simulink model "StPassCmprtMd_RfCtrl_Sw_RclRspStat"  (R2018b)
settings: Solver=FixedStepDiscrete  StartTime=0.0  StopTime=10.0  FixedStep=0.01  RelTol=1e-3
undefined symbols (not defined in the file or in its folder): KeSMSuRspStatHldTm_Val, SrcReqTp1
libraries: RspLib x20
settings Model: Creator=sn2xws  LastModifiedBy=sn2xws
settings DataIOCC: SaveFormat=StructureWithTime
settings OptimizationCC: DefaultParameterBehavior=Inlined  EnhancedBackFolding=on  PassReuseOutputArgsAs=Individual arguments  ZeroExternalMemoryAtStartup=off  ZeroInternalMemoryAtStartup=off  OptimizeBlockOrder=speed  DifferentSizesBufferReuse=on  OptimizationCustomize=off
settings DebuggingCC: ParameterTunabilityLossMsg=error
settings ModelReferenceCC: ModelReferenceNumInstancesAllowed=Single
settings SFSimCC: MATLABDynamicMemAlloc=off
settings RTWCC: SystemTargetFile=autosar.tlc  GenCodeOnly=on  TemplateMakefile=ert_default_tmf  Description=AUTOSAR  GenerateReport=on  IncludeHyperlinkInReport=on  LaunchReport=on  GenerateTraceInfo=on  GenerateTraceReport=on  GenerateTraceReportSl=on  GenerateTraceReportSf=on  GenerateTraceReportEml=on
settings CodeAppCC: ForceParamTrailComments=on  IgnoreCustomStorageClasses=off  OperatorAnnotations=on  SimulinkDataObjDesc=on  SFDataObjDesc=on  InsertBlockDesc=on
settings STFCustomTargetCC: TargetLangStandard=C99 (ISO)  MultiwordLength=256  ParMdlRefBuildCompliant=on  CompOptLevelCompliant=on  IncludeMdlTerminateFcn=off  CombineOutputUpdateFcns=on  SuppressErrorStatus=on  ERTCustomFileBanners=on  SupportNonFinite=off  SupportComplex=off  SupportContinuousTime=off  SupportNonInlinedSFcns=off  RemoveResetFunc=on  MATLABClassNameForMDSCustomization=Simulink.SoftwareTarget.ERTCustomization  AutosarCompliant=on  UseToolchainInfoCompliant=on  LookupTableObjectStructAxisOrder=2,1,3,4,...  LUTObjectStructOrderEvenSpacing=Size,Table,Breakpoints  SystemTargetFile=autosar.tlc
settings ERTTargetCC: TargetLangStandard=C99 (ISO)  ConcurrentExecutionCompliant=off  IncludeMdlTerminateFcn=off  SuppressErrorStatus=on  SupportNonFinite=off  SupportComplex=off  ModelStepFunctionPrototypeControlCompliant=off  CPPClassGenCompliant=off  AutosarCompliant=on  LookupTableObjectStructAxisOrder=2,1,3,4,...  LUTObjectStructOrderEvenSpacing=Size,Table,Breakpoints  InlinedParameterPlacement=NonHierarchical  ERTCustomFileTemplate=example_file_process.tlc

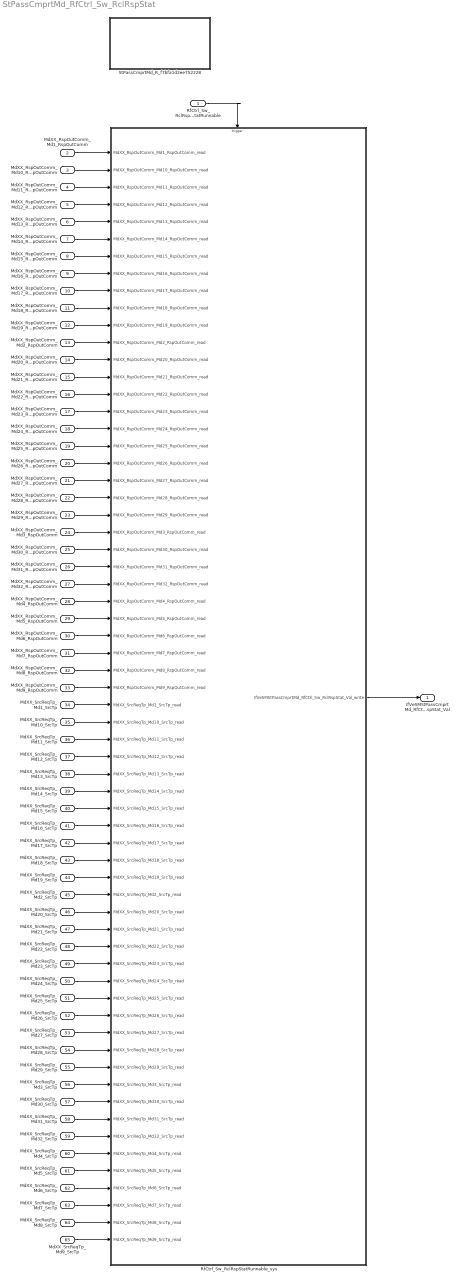
== system StPassCmprtMd_RfCtrl_Sw_RclRspStat ==
  RfCtrl_Sw_RclRspStatRunnable : Inport  SampleTime=0.01  OutputFunctionCall=on
  MdXX_RspOutComm_Md1_RspOutComm : Inport  Port=2  OutDataTypeStr=uint8  PortDimensions=1
  MdXX_RspOutComm_Md10_RspOutComm : Inport  Port=3  OutDataTypeStr=uint8  PortDimensions=1
  MdXX_RspOutComm_Md11_RspOutComm : Inport  Port=4  OutDataTypeStr=uint8  PortDimensions=1
  MdXX_RspOutComm_Md12_RspOutComm : Inport  Port=5  OutDataTypeStr=uint8  PortDimensions=1
  MdXX_RspOutComm_Md13_RspOutComm : Inport  Port=6  OutDataTypeStr=uint8  PortDimensions=1
  MdXX_RspOutComm_Md14_RspOutComm : Inport  Port=7  OutDataTypeStr=uint8  PortDimensions=1
  MdXX_RspOutComm_Md15_RspOutComm : Inport  Port=8  OutDataTypeStr=uint8  PortDimensions=1
  MdXX_RspOutComm_Md16_RspOutComm : Inport  Port=9  OutDataTypeStr=uint8  PortDimensions=1
  MdXX_RspOutComm_Md17_RspOutComm : Inport  Port=10  OutDataTypeStr=uint8  PortDimensions=1
  MdXX_RspOutComm_Md18_RspOutComm : Inport  Port=11  OutDataTypeStr=uint8  PortDimensions=1
  MdXX_RspOutComm_Md19_RspOutComm : Inport  Port=12  OutDataTypeStr=uint8  PortDimensions=1
  MdXX_RspOutComm_Md2_RspOutComm : Inport  Port=13  OutDataTypeStr=uint8  PortDimensions=1
  MdXX_RspOutComm_Md20_RspOutComm : Inport  Port=14  OutDataTypeStr=uint8  PortDimensions=1
  MdXX_RspOutComm_Md21_RspOutComm : Inport  Port=15  OutDataTypeStr=uint8  PortDimensions=1
  MdXX_RspOutComm_Md22_RspOutComm : Inport  Port=16  OutDataTypeStr=uint8  PortDimensions=1
  MdXX_RspOutComm_Md23_RspOutComm : Inport  Port=17  OutDataTypeStr=uint8  PortDimensions=1
  MdXX_RspOutComm_Md24_RspOutComm : Inport  Port=18  OutDataTypeStr=uint8  PortDimensions=1
  MdXX_RspOutComm_Md25_RspOutComm : Inport  Port=19  OutDataTypeStr=uint8  PortDimensions=1
  MdXX_RspOutComm_Md26_RspOutComm : Inport  Port=20  OutDataTypeStr=uint8  PortDimensions=1
  MdXX_RspOutComm_Md27_RspOutComm : Inport  Port=21  OutDataTypeStr=uint8  PortDimensions=1
  MdXX_RspOutComm_Md28_RspOutComm : Inport  Port=22  OutDataTypeStr=uint8  PortDimensions=1
  MdXX_RspOutComm_Md29_RspOutComm : Inport  Port=23  OutDataTypeStr=uint8  PortDimensions=1
  MdXX_RspOutComm_Md3_RspOutComm : Inport  Port=24  OutDataTypeStr=uint8  PortDimensions=1
  MdXX_RspOutComm_Md30_RspOutComm : Inport  Port=25  OutDataTypeStr=uint8  PortDimensions=1
  MdXX_RspOutComm_Md31_RspOutComm : Inport  Port=26  OutDataTypeStr=uint8  PortDimensions=1
  MdXX_RspOutComm_Md32_RspOutComm : Inport  Port=27  OutDataTypeStr=uint8  PortDimensions=1
  MdXX_RspOutComm_Md4_RspOutComm : Inport  Port=28  OutDataTypeStr=uint8  PortDimensions=1
  MdXX_RspOutComm_Md5_RspOutComm : Inport  Port=29  OutDataTypeStr=uint8  PortDimensions=1
  MdXX_RspOutComm_Md6_RspOutComm : Inport  Port=30  OutDataTypeStr=uint8  PortDimensions=1
  MdXX_RspOutComm_Md7_RspOutComm : Inport  Port=31  OutDataTypeStr=uint8  PortDimensions=1
  MdXX_RspOutComm_Md8_RspOutComm : Inport  Port=32  OutDataTypeStr=uint8  PortDimensions=1
  MdXX_RspOutComm_Md9_RspOutComm : Inport  Port=33  OutDataTypeStr=uint8  PortDimensions=1
  MdXX_SrcReqTp_Md1_SrcTp : Inport  Port=34  OutDataTypeStr=Enum: SrcReqTp1  PortDimensions=1
  MdXX_SrcReqTp_Md10_SrcTp : Inport  Port=35  OutDataTypeStr=Enum: SrcReqTp1  PortDimensions=1
  MdXX_SrcReqTp_Md11_SrcTp : Inport  Port=36  OutDataTypeStr=Enum: SrcReqTp1  PortDimensions=1
  MdXX_SrcReqTp_Md12_SrcTp : Inport  Port=37  OutDataTypeStr=Enum: SrcReqTp1  PortDimensions=1
  MdXX_SrcReqTp_Md13_SrcTp : Inport  Port=38  OutDataTypeStr=Enum: SrcReqTp1  PortDimensions=1
  MdXX_SrcReqTp_Md14_SrcTp : Inport  Port=39  OutDataTypeStr=Enum: SrcReqTp1  PortDimensions=1
  MdXX_SrcReqTp_Md15_SrcTp : Inport  Port=40  OutDataTypeStr=Enum: SrcReqTp1  PortDimensions=1
  MdXX_SrcReqTp_Md16_SrcTp : Inport  Port=41  OutDataTypeStr=Enum: SrcReqTp1  PortDimensions=1
  MdXX_SrcReqTp_Md17_SrcTp : Inport  Port=42  OutDataTypeStr=Enum: SrcReqTp1  PortDimensions=1
  MdXX_SrcReqTp_Md18_SrcTp : Inport  Port=43  OutDataTypeStr=Enum: SrcReqTp1  PortDimensions=1
  MdXX_SrcReqTp_Md19_SrcTp : Inport  Port=44  OutDataTypeStr=Enum: SrcReqTp1  PortDimensions=1
  MdXX_SrcReqTp_Md2_SrcTp : Inport  Port=45  OutDataTypeStr=Enum: SrcReqTp1  PortDimensions=1
  MdXX_SrcReqTp_Md20_SrcTp : Inport  Port=46  OutDataTypeStr=Enum: SrcReqTp1  PortDimensions=1
  MdXX_SrcReqTp_Md21_SrcTp : Inport  Port=47  OutDataTypeStr=Enum: SrcReqTp1  PortDimensions=1
  MdXX_SrcReqTp_Md22_SrcTp : Inport  Port=48  OutDataTypeStr=Enum: SrcReqTp1  PortDimensions=1
  MdXX_SrcReqTp_Md23_SrcTp : Inport  Port=49  OutDataTypeStr=Enum: SrcReqTp1  PortDimensions=1
  MdXX_SrcReqTp_Md24_SrcTp : Inport  Port=50  OutDataTypeStr=Enum: SrcReqTp1  PortDimensions=1
  MdXX_SrcReqTp_Md25_SrcTp : Inport  Port=51  OutDataTypeStr=Enum: SrcReqTp1  PortDimensions=1
  MdXX_SrcReqTp_Md26_SrcTp : Inport  Port=52  OutDataTypeStr=Enum: SrcReqTp1  PortDimensions=1
  MdXX_SrcReqTp_Md27_SrcTp : Inport  Port=53  OutDataTypeStr=Enum: SrcReqTp1  PortDimensions=1
  MdXX_SrcReqTp_Md28_SrcTp : Inport  Port=54  OutDataTypeStr=Enum: SrcReqTp1  PortDimensions=1
  MdXX_SrcReqTp_Md29_SrcTp : Inport  Port=55  OutDataTypeStr=Enum: SrcReqTp1  PortDimensions=1
  MdXX_SrcReqTp_Md3_SrcTp : Inport  Port=56  OutDataTypeStr=Enum: SrcReqTp1  PortDimensions=1
  MdXX_SrcReqTp_Md30_SrcTp : Inport  Port=57  OutDataTypeStr=Enum: SrcReqTp1  PortDimensions=1
  MdXX_SrcReqTp_Md31_SrcTp : Inport  Port=58  OutDataTypeStr=Enum: SrcReqTp1  PortDimensions=1
  MdXX_SrcReqTp_Md32_SrcTp : Inport  Port=59  OutDataTypeStr=Enum: SrcReqTp1  PortDimensions=1
  MdXX_SrcReqTp_Md4_SrcTp : Inport  Port=60  OutDataTypeStr=Enum: SrcReqTp1  PortDimensions=1
  MdXX_SrcReqTp_Md5_SrcTp : Inport  Port=61  OutDataTypeStr=Enum: SrcReqTp1  PortDimensions=1
  MdXX_SrcReqTp_Md6_SrcTp : Inport  Port=62  OutDataTypeStr=Enum: SrcReqTp1  PortDimensions=1
  MdXX_SrcReqTp_Md7_SrcTp : Inport  Port=63  OutDataTypeStr=Enum: SrcReqTp1  PortDimensions=1
  MdXX_SrcReqTp_Md8_SrcTp : Inport  Port=64  OutDataTypeStr=Enum: SrcReqTp1  PortDimensions=1
  MdXX_SrcReqTp_Md9_SrcTp : Inport  Port=65  OutDataTypeStr=Enum: SrcReqTp1  PortDimensions=1
  RfCtrl_Sw_RclRspStatRunnable_sys : Subsystem
  StPassCmprtMd_R_f7bfa1d2ee752228 : Subsystem
  IfVeSMStPassCmprtMd_RfCtrl_Sw_RclRspStat_Val : Outport  OutDataTypeStr=uint8  PortDimensions=1
  wires:
  MdXX_RspOutComm_Md1_RspOutComm/1 -> RfCtrl_Sw_RclRspStatRunnable_sys/1(MdXX_RspOutComm_Md1_RspOutComm_read)
  MdXX_RspOutComm_Md10_RspOutComm/1 -> RfCtrl_Sw_RclRspStatRunnable_sys/2(MdXX_RspOutComm_Md10_RspOutComm_read)
  MdXX_RspOutComm_Md11_RspOutComm/1 -> RfCtrl_Sw_RclRspStatRunnable_sys/3(MdXX_RspOutComm_Md11_RspOutComm_read)
  MdXX_RspOutComm_Md12_RspOutComm/1 -> RfCtrl_Sw_RclRspStatRunnable_sys/4(MdXX_RspOutComm_Md12_RspOutComm_read)
  MdXX_RspOutComm_Md13_RspOutComm/1 -> RfCtrl_Sw_RclRspStatRunnable_sys/5(MdXX_RspOutComm_Md13_RspOutComm_read)
  MdXX_RspOutComm_Md14_RspOutComm/1 -> RfCtrl_Sw_RclRspStatRunnable_sys/6(MdXX_RspOutComm_Md14_RspOutComm_read)
  MdXX_RspOutComm_Md15_RspOutComm/1 -> RfCtrl_Sw_RclRspStatRunnable_sys/7(MdXX_RspOutComm_Md15_RspOutComm_read)
  MdXX_RspOutComm_Md16_RspOutComm/1 -> RfCtrl_Sw_RclRspStatRunnable_sys/8(MdXX_RspOutComm_Md16_RspOutComm_read)
  MdXX_RspOutComm_Md17_RspOutComm/1 -> RfCtrl_Sw_RclRspStatRunnable_sys/9(MdXX_RspOutComm_Md17_RspOutComm_read)
  MdXX_RspOutComm_Md18_RspOutComm/1 -> RfCtrl_Sw_RclRspStatRunnable_sys/10(MdXX_RspOutComm_Md18_RspOutComm_read)
  MdXX_RspOutComm_Md19_RspOutComm/1 -> RfCtrl_Sw_RclRspStatRunnable_sys/11(MdXX_RspOutComm_Md19_RspOutComm_read)
  MdXX_RspOutComm_Md2_RspOutComm/1 -> RfCtrl_Sw_RclRspStatRunnable_sys/12(MdXX_RspOutComm_Md2_RspOutComm_read)
  MdXX_RspOutComm_Md20_RspOutComm/1 -> RfCtrl_Sw_RclRspStatRunnable_sys/13(MdXX_RspOutComm_Md20_RspOutComm_read)
  MdXX_RspOutComm_Md21_RspOutComm/1 -> RfCtrl_Sw_RclRspStatRunnable_sys/14(MdXX_RspOutComm_Md21_RspOutComm_read)
  MdXX_RspOutComm_Md22_RspOutComm/1 -> RfCtrl_Sw_RclRspStatRunnable_sys/15(MdXX_RspOutComm_Md22_RspOutComm_read)
  MdXX_RspOutComm_Md23_RspOutComm/1 -> RfCtrl_Sw_RclRspStatRunnable_sys/16(MdXX_RspOutComm_Md23_RspOutComm_read)
  MdXX_RspOutComm_Md24_RspOutComm/1 -> RfCtrl_Sw_RclRspStatRunnable_sys/17(MdXX_RspOutComm_Md24_RspOutComm_read)
  MdXX_RspOutComm_Md25_RspOutComm/1 -> RfCtrl_Sw_RclRspStatRunnable_sys/18(MdXX_RspOutComm_Md25_RspOutComm_read)
  MdXX_RspOutComm_Md26_RspOutComm/1 -> RfCtrl_Sw_RclRspStatRunnable_sys/19(MdXX_RspOutComm_Md26_RspOutComm_read)
  MdXX_RspOutComm_Md27_RspOutComm/1 -> RfCtrl_Sw_RclRspStatRunnable_sys/20(MdXX_RspOutComm_Md27_RspOutComm_read)
  MdXX_RspOutComm_Md28_RspOutComm/1 -> RfCtrl_Sw_RclRspStatRunnable_sys/21(MdXX_RspOutComm_Md28_RspOutComm_read)
  MdXX_RspOutComm_Md29_RspOutComm/1 -> RfCtrl_Sw_RclRspStatRunnable_sys/22(MdXX_RspOutComm_Md29_RspOutComm_read)
  MdXX_RspOutComm_Md3_RspOutComm/1 -> RfCtrl_Sw_RclRspStatRunnable_sys/23(MdXX_RspOutComm_Md3_RspOutComm_read)
  MdXX_RspOutComm_Md30_RspOutComm/1 -> RfCtrl_Sw_RclRspStatRunnable_sys/24(MdXX_RspOutComm_Md30_RspOutComm_read)
  MdXX_RspOutComm_Md31_RspOutComm/1 -> RfCtrl_Sw_RclRspStatRunnable_sys/25(MdXX_RspOutComm_Md31_RspOutComm_read)
  MdXX_RspOutComm_Md32_RspOutComm/1 -> RfCtrl_Sw_RclRspStatRunnable_sys/26(MdXX_RspOutComm_Md32_RspOutComm_read)
  MdXX_RspOutComm_Md4_RspOutComm/1 -> RfCtrl_Sw_RclRspStatRunnable_sys/27(MdXX_RspOutComm_Md4_RspOutComm_read)
  MdXX_RspOutComm_Md5_RspOutComm/1 -> RfCtrl_Sw_RclRspStatRunnable_sys/28(MdXX_RspOutComm_Md5_RspOutComm_read)
  MdXX_RspOutComm_Md6_RspOutComm/1 -> RfCtrl_Sw_RclRspStatRunnable_sys/29(MdXX_RspOutComm_Md6_RspOutComm_read)
  MdXX_RspOutComm_Md7_RspOutComm/1 -> RfCtrl_Sw_RclRspStatRunnable_sys/30(MdXX_RspOutComm_Md7_RspOutComm_read)
  MdXX_RspOutComm_Md8_RspOutComm/1 -> RfCtrl_Sw_RclRspStatRunnable_sys/31(MdXX_RspOutComm_Md8_RspOutComm_read)
  MdXX_RspOutComm_Md9_RspOutComm/1 -> RfCtrl_Sw_RclRspStatRunnable_sys/32(MdXX_RspOutComm_Md9_RspOutComm_read)
  MdXX_SrcReqTp_Md1_SrcTp/1 -> RfCtrl_Sw_RclRspStatRunnable_sys/33(MdXX_SrcReqTp_Md1_SrcTp_read)
  MdXX_SrcReqTp_Md10_SrcTp/1 -> RfCtrl_Sw_RclRspStatRunnable_sys/34(MdXX_SrcReqTp_Md10_SrcTp_read)
  MdXX_SrcReqTp_Md11_SrcTp/1 -> RfCtrl_Sw_RclRspStatRunnable_sys/35(MdXX_SrcReqTp_Md11_SrcTp_read)
  MdXX_SrcReqTp_Md12_SrcTp/1 -> RfCtrl_Sw_RclRspStatRunnable_sys/36(MdXX_SrcReqTp_Md12_SrcTp_read)
  MdXX_SrcReqTp_Md13_SrcTp/1 -> RfCtrl_Sw_RclRspStatRunnable_sys/37(MdXX_SrcReqTp_Md13_SrcTp_read)
  MdXX_SrcReqTp_Md14_SrcTp/1 -> RfCtrl_Sw_RclRspStatRunnable_sys/38(MdXX_SrcReqTp_Md14_SrcTp_read)
  MdXX_SrcReqTp_Md15_SrcTp/1 -> RfCtrl_Sw_RclRspStatRunnable_sys/39(MdXX_SrcReqTp_Md15_SrcTp_read)
  MdXX_SrcReqTp_Md16_SrcTp/1 -> RfCtrl_Sw_RclRspStatRunnable_sys/40(MdXX_SrcReqTp_Md16_SrcTp_read)
  MdXX_SrcReqTp_Md17_SrcTp/1 -> RfCtrl_Sw_RclRspStatRunnable_sys/41(MdXX_SrcReqTp_Md17_SrcTp_read)
  MdXX_SrcReqTp_Md18_SrcTp/1 -> RfCtrl_Sw_RclRspStatRunnable_sys/42(MdXX_SrcReqTp_Md18_SrcTp_read)
  MdXX_SrcReqTp_Md19_SrcTp/1 -> RfCtrl_Sw_RclRspStatRunnable_sys/43(MdXX_SrcReqTp_Md19_SrcTp_read)
  MdXX_SrcReqTp_Md2_SrcTp/1 -> RfCtrl_Sw_RclRspStatRunnable_sys/44(MdXX_SrcReqTp_Md2_SrcTp_read)
  MdXX_SrcReqTp_Md20_SrcTp/1 -> RfCtrl_Sw_RclRspStatRunnable_sys/45(MdXX_SrcReqTp_Md20_SrcTp_read)
  MdXX_SrcReqTp_Md21_SrcTp/1 -> RfCtrl_Sw_RclRspStatRunnable_sys/46(MdXX_SrcReqTp_Md21_SrcTp_read)
  MdXX_SrcReqTp_Md22_SrcTp/1 -> RfCtrl_Sw_RclRspStatRunnable_sys/47(MdXX_SrcReqTp_Md22_SrcTp_read)
  MdXX_SrcReqTp_Md23_SrcTp/1 -> RfCtrl_Sw_RclRspStatRunnable_sys/48(MdXX_SrcReqTp_Md23_SrcTp_read)
  MdXX_SrcReqTp_Md24_SrcTp/1 -> RfCtrl_Sw_RclRspStatRunnable_sys/49(MdXX_SrcReqTp_Md24_SrcTp_read)
  MdXX_SrcReqTp_Md25_SrcTp/1 -> RfCtrl_Sw_RclRspStatRunnable_sys/50(MdXX_SrcReqTp_Md25_SrcTp_read)
  MdXX_SrcReqTp_Md26_SrcTp/1 -> RfCtrl_Sw_RclRspStatRunnable_sys/51(MdXX_SrcReqTp_Md26_SrcTp_read)
  MdXX_SrcReqTp_Md27_SrcTp/1 -> RfCtrl_Sw_RclRspStatRunnable_sys/52(MdXX_SrcReqTp_Md27_SrcTp_read)
  MdXX_SrcReqTp_Md28_SrcTp/1 -> RfCtrl_Sw_RclRspStatRunnable_sys/53(MdXX_SrcReqTp_Md28_SrcTp_read)
  MdXX_SrcReqTp_Md29_SrcTp/1 -> RfCtrl_Sw_RclRspStatRunnable_sys/54(MdXX_SrcReqTp_Md29_SrcTp_read)
  MdXX_SrcReqTp_Md3_SrcTp/1 -> RfCtrl_Sw_RclRspStatRunnable_sys/55(MdXX_SrcReqTp_Md3_SrcTp_read)
  MdXX_SrcReqTp_Md30_SrcTp/1 -> RfCtrl_Sw_RclRspStatRunnable_sys/56(MdXX_SrcReqTp_Md30_SrcTp_read)
  MdXX_SrcReqTp_Md31_SrcTp/1 -> RfCtrl_Sw_RclRspStatRunnable_sys/57(MdXX_SrcReqTp_Md31_SrcTp_read)
  MdXX_SrcReqTp_Md32_SrcTp/1 -> RfCtrl_Sw_RclRspStatRunnable_sys/58(MdXX_SrcReqTp_Md32_SrcTp_read)
  MdXX_SrcReqTp_Md4_SrcTp/1 -> RfCtrl_Sw_RclRspStatRunnable_sys/59(MdXX_SrcReqTp_Md4_SrcTp_read)
  MdXX_SrcReqTp_Md5_SrcTp/1 -> RfCtrl_Sw_RclRspStatRunnable_sys/60(MdXX_SrcReqTp_Md5_SrcTp_read)
  MdXX_SrcReqTp_Md6_SrcTp/1 -> RfCtrl_Sw_RclRspStatRunnable_sys/61(MdXX_SrcReqTp_Md6_SrcTp_read)
  MdXX_SrcReqTp_Md7_SrcTp/1 -> RfCtrl_Sw_RclRspStatRunnable_sys/62(MdXX_SrcReqTp_Md7_SrcTp_read)
  MdXX_SrcReqTp_Md8_SrcTp/1 -> RfCtrl_Sw_RclRspStatRunnable_sys/63(MdXX_SrcReqTp_Md8_SrcTp_read)
  MdXX_SrcReqTp_Md9_SrcTp/1 -> RfCtrl_Sw_RclRspStatRunnable_sys/64(MdXX_SrcReqTp_Md9_SrcTp_read)
  RfCtrl_Sw_RclRspStatRunnable_sys/1(IfVeSMStPassCmprtMd_RfCtrl_Sw_RclRspStat_Val_write) -> IfVeSMStPassCmprtMd_RfCtrl_Sw_RclRspStat_Val/1
  RfCtrl_Sw_RclRspStatRunnable/1 -> RfCtrl_Sw_RclRspStatRunnable_sys/Trigger

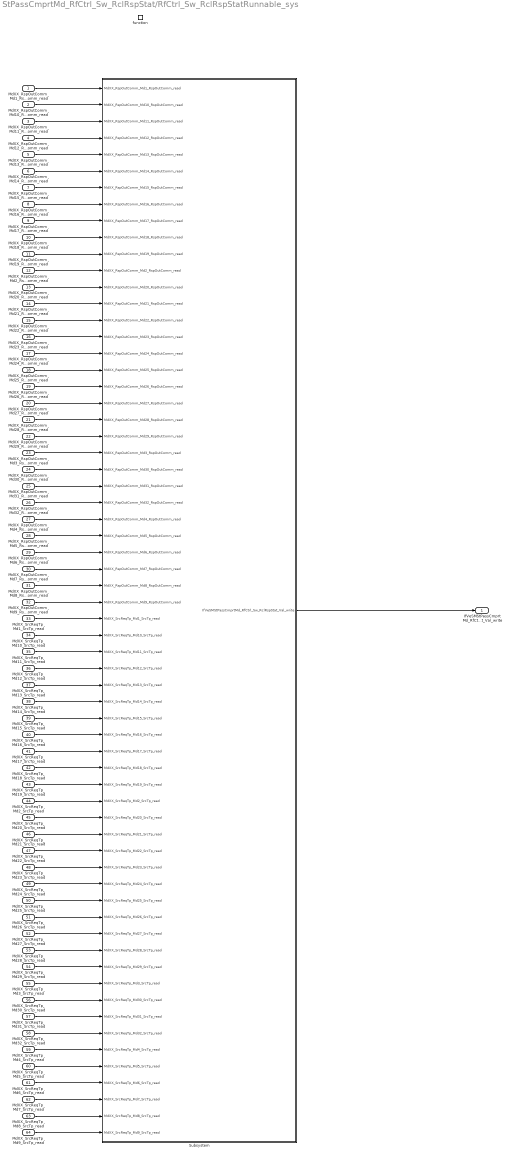
== system StPassCmprtMd_RfCtrl_Sw_RclRspStat/RfCtrl_Sw_RclRspStatRunnable_sys ==
  MdXX_RspOutComm_Md1_RspOutComm_read : Inport
  MdXX_RspOutComm_Md10_RspOutComm_read : Inport  Port=2
  MdXX_RspOutComm_Md11_RspOutComm_read : Inport  Port=3
  MdXX_RspOutComm_Md12_RspOutComm_read : Inport  Port=4
  MdXX_RspOutComm_Md13_RspOutComm_read : Inport  Port=5
  MdXX_RspOutComm_Md14_RspOutComm_read : Inport  Port=6
  MdXX_RspOutComm_Md15_RspOutComm_read : Inport  Port=7
  MdXX_RspOutComm_Md16_RspOutComm_read : Inport  Port=8
  MdXX_RspOutComm_Md17_RspOutComm_read : Inport  Port=9
  MdXX_RspOutComm_Md18_RspOutComm_read : Inport  Port=10
  MdXX_RspOutComm_Md19_RspOutComm_read : Inport  Port=11
  MdXX_RspOutComm_Md2_RspOutComm_read : Inport  Port=12
  MdXX_RspOutComm_Md20_RspOutComm_read : Inport  Port=13
  MdXX_RspOutComm_Md21_RspOutComm_read : Inport  Port=14
  MdXX_RspOutComm_Md22_RspOutComm_read : Inport  Port=15
  MdXX_RspOutComm_Md23_RspOutComm_read : Inport  Port=16
  MdXX_RspOutComm_Md24_RspOutComm_read : Inport  Port=17
  MdXX_RspOutComm_Md25_RspOutComm_read : Inport  Port=18
  MdXX_RspOutComm_Md26_RspOutComm_read : Inport  Port=19
  MdXX_RspOutComm_Md27_RspOutComm_read : Inport  Port=20
  MdXX_RspOutComm_Md28_RspOutComm_read : Inport  Port=21
  MdXX_RspOutComm_Md29_RspOutComm_read : Inport  Port=22
  MdXX_RspOutComm_Md3_RspOutComm_read : Inport  Port=23
  MdXX_RspOutComm_Md30_RspOutComm_read : Inport  Port=24
  MdXX_RspOutComm_Md31_RspOutComm_read : Inport  Port=25
  MdXX_RspOutComm_Md32_RspOutComm_read : Inport  Port=26
  MdXX_RspOutComm_Md4_RspOutComm_read : Inport  Port=27
  MdXX_RspOutComm_Md5_RspOutComm_read : Inport  Port=28
  MdXX_RspOutComm_Md6_RspOutComm_read : Inport  Port=29
  MdXX_RspOutComm_Md7_RspOutComm_read : Inport  Port=30
  MdXX_RspOutComm_Md8_RspOutComm_read : Inport  Port=31
  MdXX_RspOutComm_Md9_RspOutComm_read : Inport  Port=32
  MdXX_SrcReqTp_Md1_SrcTp_read : Inport  Port=33
  MdXX_SrcReqTp_Md10_SrcTp_read : Inport  Port=34
  MdXX_SrcReqTp_Md11_SrcTp_read : Inport  Port=35
  MdXX_SrcReqTp_Md12_SrcTp_read : Inport  Port=36
  MdXX_SrcReqTp_Md13_SrcTp_read : Inport  Port=37
  MdXX_SrcReqTp_Md14_SrcTp_read : Inport  Port=38
  MdXX_SrcReqTp_Md15_SrcTp_read : Inport  Port=39
  MdXX_SrcReqTp_Md16_SrcTp_read : Inport  Port=40
  MdXX_SrcReqTp_Md17_SrcTp_read : Inport  Port=41
  MdXX_SrcReqTp_Md18_SrcTp_read : Inport  Port=42
  MdXX_SrcReqTp_Md19_SrcTp_read : Inport  Port=43
  MdXX_SrcReqTp_Md2_SrcTp_read : Inport  Port=44
  MdXX_SrcReqTp_Md20_SrcTp_read : Inport  Port=45
  MdXX_SrcReqTp_Md21_SrcTp_read : Inport  Port=46
  MdXX_SrcReqTp_Md22_SrcTp_read : Inport  Port=47
  MdXX_SrcReqTp_Md23_SrcTp_read : Inport  Port=48
  MdXX_SrcReqTp_Md24_SrcTp_read : Inport  Port=49
  MdXX_SrcReqTp_Md25_SrcTp_read : Inport  Port=50
  MdXX_SrcReqTp_Md26_SrcTp_read : Inport  Port=51
  MdXX_SrcReqTp_Md27_SrcTp_read : Inport  Port=52
  MdXX_SrcReqTp_Md28_SrcTp_read : Inport  Port=53
  MdXX_SrcReqTp_Md29_SrcTp_read : Inport  Port=54
  MdXX_SrcReqTp_Md3_SrcTp_read : Inport  Port=55
  MdXX_SrcReqTp_Md30_SrcTp_read : Inport  Port=56
  MdXX_SrcReqTp_Md31_SrcTp_read : Inport  Port=57
  MdXX_SrcReqTp_Md32_SrcTp_read : Inport  Port=58
  MdXX_SrcReqTp_Md4_SrcTp_read : Inport  Port=59
  MdXX_SrcReqTp_Md5_SrcTp_read : Inport  Port=60
  MdXX_SrcReqTp_Md6_SrcTp_read : Inport  Port=61
  MdXX_SrcReqTp_Md7_SrcTp_read : Inport  Port=62
  MdXX_SrcReqTp_Md8_SrcTp_read : Inport  Port=63
  MdXX_SrcReqTp_Md9_SrcTp_read : Inport  Port=64
  function : TriggerPort  TriggerType=function-call  VariantControl=(inherit)  SampleTimeType=periodic  SampleTime=-1
  Subsystem : Subsystem
  IfVeSMStPassCmprtMd_RfCtrl_Sw_RclRspStat_Val_write : Outport
      settings: EnsureOutportIsVirtual=on
  wires:
  MdXX_RspOutComm_Md1_RspOutComm_read/1 -> Subsystem/1(MdXX_RspOutComm_Md1_RspOutComm_read)
  MdXX_RspOutComm_Md10_RspOutComm_read/1 -> Subsystem/2(MdXX_RspOutComm_Md10_RspOutComm_read)
  MdXX_RspOutComm_Md11_RspOutComm_read/1 -> Subsystem/3(MdXX_RspOutComm_Md11_RspOutComm_read)
  MdXX_RspOutComm_Md12_RspOutComm_read/1 -> Subsystem/4(MdXX_RspOutComm_Md12_RspOutComm_read)
  MdXX_RspOutComm_Md13_RspOutComm_read/1 -> Subsystem/5(MdXX_RspOutComm_Md13_RspOutComm_read)
  MdXX_RspOutComm_Md14_RspOutComm_read/1 -> Subsystem/6(MdXX_RspOutComm_Md14_RspOutComm_read)
  MdXX_RspOutComm_Md15_RspOutComm_read/1 -> Subsystem/7(MdXX_RspOutComm_Md15_RspOutComm_read)
  MdXX_RspOutComm_Md16_RspOutComm_read/1 -> Subsystem/8(MdXX_RspOutComm_Md16_RspOutComm_read)
  MdXX_RspOutComm_Md17_RspOutComm_read/1 -> Subsystem/9(MdXX_RspOutComm_Md17_RspOutComm_read)
  MdXX_RspOutComm_Md18_RspOutComm_read/1 -> Subsystem/10(MdXX_RspOutComm_Md18_RspOutComm_read)
  MdXX_RspOutComm_Md19_RspOutComm_read/1 -> Subsystem/11(MdXX_RspOutComm_Md19_RspOutComm_read)
  MdXX_RspOutComm_Md2_RspOutComm_read/1 -> Subsystem/12(MdXX_RspOutComm_Md2_RspOutComm_read)
  MdXX_RspOutComm_Md20_RspOutComm_read/1 -> Subsystem/13(MdXX_RspOutComm_Md20_RspOutComm_read)
  MdXX_RspOutComm_Md21_RspOutComm_read/1 -> Subsystem/14(MdXX_RspOutComm_Md21_RspOutComm_read)
  MdXX_RspOutComm_Md22_RspOutComm_read/1 -> Subsystem/15(MdXX_RspOutComm_Md22_RspOutComm_read)
  MdXX_RspOutComm_Md23_RspOutComm_read/1 -> Subsystem/16(MdXX_RspOutComm_Md23_RspOutComm_read)
  MdXX_RspOutComm_Md24_RspOutComm_read/1 -> Subsystem/17(MdXX_RspOutComm_Md24_RspOutComm_read)
  MdXX_RspOutComm_Md25_RspOutComm_read/1 -> Subsystem/18(MdXX_RspOutComm_Md25_RspOutComm_read)
  MdXX_RspOutComm_Md26_RspOutComm_read/1 -> Subsystem/19(MdXX_RspOutComm_Md26_RspOutComm_read)
  MdXX_RspOutComm_Md27_RspOutComm_read/1 -> Subsystem/20(MdXX_RspOutComm_Md27_RspOutComm_read)
  MdXX_RspOutComm_Md28_RspOutComm_read/1 -> Subsystem/21(MdXX_RspOutComm_Md28_RspOutComm_read)
  MdXX_RspOutComm_Md29_RspOutComm_read/1 -> Subsystem/22(MdXX_RspOutComm_Md29_RspOutComm_read)
  MdXX_RspOutComm_Md3_RspOutComm_read/1 -> Subsystem/23(MdXX_RspOutComm_Md3_RspOutComm_read)
  MdXX_RspOutComm_Md30_RspOutComm_read/1 -> Subsystem/24(MdXX_RspOutComm_Md30_RspOutComm_read)
  MdXX_RspOutComm_Md31_RspOutComm_read/1 -> Subsystem/25(MdXX_RspOutComm_Md31_RspOutComm_read)
  MdXX_RspOutComm_Md32_RspOutComm_read/1 -> Subsystem/26(MdXX_RspOutComm_Md32_RspOutComm_read)
  MdXX_RspOutComm_Md4_RspOutComm_read/1 -> Subsystem/27(MdXX_RspOutComm_Md4_RspOutComm_read)
  MdXX_RspOutComm_Md5_RspOutComm_read/1 -> Subsystem/28(MdXX_RspOutComm_Md5_RspOutComm_read)
  MdXX_RspOutComm_Md6_RspOutComm_read/1 -> Subsystem/29(MdXX_RspOutComm_Md6_RspOutComm_read)
  MdXX_RspOutComm_Md7_RspOutComm_read/1 -> Subsystem/30(MdXX_RspOutComm_Md7_RspOutComm_read)
  MdXX_RspOutComm_Md8_RspOutComm_read/1 -> Subsystem/31(MdXX_RspOutComm_Md8_RspOutComm_read)
  MdXX_RspOutComm_Md9_RspOutComm_read/1 -> Subsystem/32(MdXX_RspOutComm_Md9_RspOutComm_read)
  MdXX_SrcReqTp_Md1_SrcTp_read/1 -> Subsystem/33(MdXX_SrcReqTp_Md1_SrcTp_read)
  MdXX_SrcReqTp_Md10_SrcTp_read/1 -> Subsystem/34(MdXX_SrcReqTp_Md10_SrcTp_read)
  MdXX_SrcReqTp_Md11_SrcTp_read/1 -> Subsystem/35(MdXX_SrcReqTp_Md11_SrcTp_read)
  MdXX_SrcReqTp_Md12_SrcTp_read/1 -> Subsystem/36(MdXX_SrcReqTp_Md12_SrcTp_read)
  MdXX_SrcReqTp_Md13_SrcTp_read/1 -> Subsystem/37(MdXX_SrcReqTp_Md13_SrcTp_read)
  MdXX_SrcReqTp_Md14_SrcTp_read/1 -> Subsystem/38(MdXX_SrcReqTp_Md14_SrcTp_read)
  MdXX_SrcReqTp_Md15_SrcTp_read/1 -> Subsystem/39(MdXX_SrcReqTp_Md15_SrcTp_read)
  MdXX_SrcReqTp_Md16_SrcTp_read/1 -> Subsystem/40(MdXX_SrcReqTp_Md16_SrcTp_read)
  MdXX_SrcReqTp_Md17_SrcTp_read/1 -> Subsystem/41(MdXX_SrcReqTp_Md17_SrcTp_read)
  MdXX_SrcReqTp_Md18_SrcTp_read/1 -> Subsystem/42(MdXX_SrcReqTp_Md18_SrcTp_read)
  MdXX_SrcReqTp_Md19_SrcTp_read/1 -> Subsystem/43(MdXX_SrcReqTp_Md19_SrcTp_read)
  MdXX_SrcReqTp_Md2_SrcTp_read/1 -> Subsystem/44(MdXX_SrcReqTp_Md2_SrcTp_read)
  MdXX_SrcReqTp_Md20_SrcTp_read/1 -> Subsystem/45(MdXX_SrcReqTp_Md20_SrcTp_read)
  MdXX_SrcReqTp_Md21_SrcTp_read/1 -> Subsystem/46(MdXX_SrcReqTp_Md21_SrcTp_read)
  MdXX_SrcReqTp_Md22_SrcTp_read/1 -> Subsystem/47(MdXX_SrcReqTp_Md22_SrcTp_read)
  MdXX_SrcReqTp_Md23_SrcTp_read/1 -> Subsystem/48(MdXX_SrcReqTp_Md23_SrcTp_read)
  MdXX_SrcReqTp_Md24_SrcTp_read/1 -> Subsystem/49(MdXX_SrcReqTp_Md24_SrcTp_read)
  MdXX_SrcReqTp_Md25_SrcTp_read/1 -> Subsystem/50(MdXX_SrcReqTp_Md25_SrcTp_read)
  MdXX_SrcReqTp_Md26_SrcTp_read/1 -> Subsystem/51(MdXX_SrcReqTp_Md26_SrcTp_read)
  MdXX_SrcReqTp_Md27_SrcTp_read/1 -> Subsystem/52(MdXX_SrcReqTp_Md27_SrcTp_read)
  MdXX_SrcReqTp_Md28_SrcTp_read/1 -> Subsystem/53(MdXX_SrcReqTp_Md28_SrcTp_read)
  MdXX_SrcReqTp_Md29_SrcTp_read/1 -> Subsystem/54(MdXX_SrcReqTp_Md29_SrcTp_read)
  MdXX_SrcReqTp_Md3_SrcTp_read/1 -> Subsystem/55(MdXX_SrcReqTp_Md3_SrcTp_read)
  MdXX_SrcReqTp_Md30_SrcTp_read/1 -> Subsystem/56(MdXX_SrcReqTp_Md30_SrcTp_read)
  MdXX_SrcReqTp_Md31_SrcTp_read/1 -> Subsystem/57(MdXX_SrcReqTp_Md31_SrcTp_read)
  MdXX_SrcReqTp_Md32_SrcTp_read/1 -> Subsystem/58(MdXX_SrcReqTp_Md32_SrcTp_read)
  MdXX_SrcReqTp_Md4_SrcTp_read/1 -> Subsystem/59(MdXX_SrcReqTp_Md4_SrcTp_read)
  MdXX_SrcReqTp_Md5_SrcTp_read/1 -> Subsystem/60(MdXX_SrcReqTp_Md5_SrcTp_read)
  MdXX_SrcReqTp_Md6_SrcTp_read/1 -> Subsystem/61(MdXX_SrcReqTp_Md6_SrcTp_read)
  MdXX_SrcReqTp_Md7_SrcTp_read/1 -> Subsystem/62(MdXX_SrcReqTp_Md7_SrcTp_read)
  MdXX_SrcReqTp_Md8_SrcTp_read/1 -> Subsystem/63(MdXX_SrcReqTp_Md8_SrcTp_read)
  MdXX_SrcReqTp_Md9_SrcTp_read/1 -> Subsystem/64(MdXX_SrcReqTp_Md9_SrcTp_read)
  Subsystem/1(IfVeSMStPassCmprtMd_RfCtrl_Sw_RclRspStat_Val_write) -> IfVeSMStPassCmprtMd_RfCtrl_Sw_RclRspStat_Val_write/1

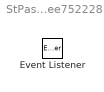
== system StPassCmprtMd_RfCtrl_Sw_RclRspStat/StPassCmprtMd_R_f7bfa1d2ee752228 ==
  Event Listener : EventListener  EventName=reset

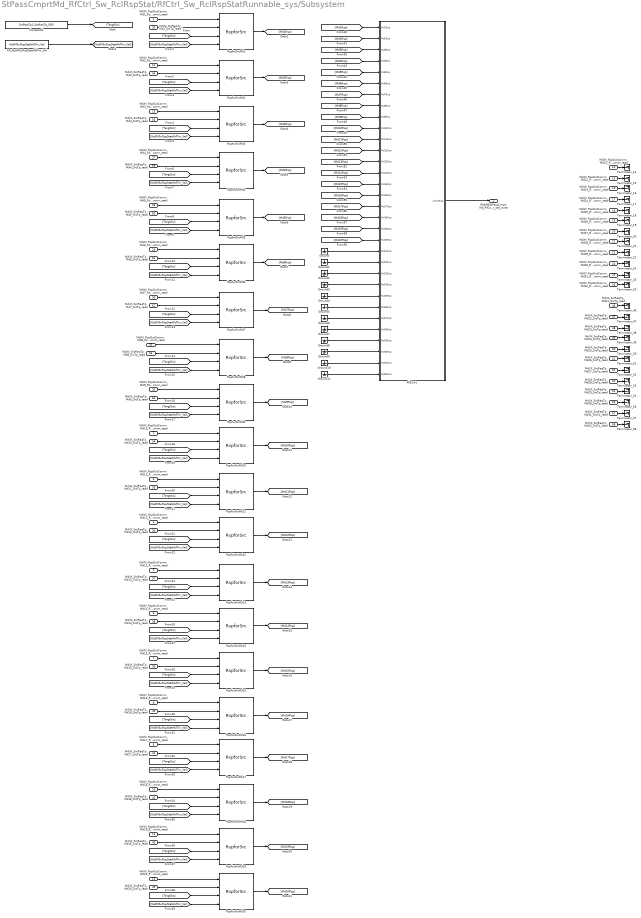
== system StPassCmprtMd_RfCtrl_Sw_RclRspStat/RfCtrl_Sw_RclRspStatRunnable_sys/Subsystem ==
  MdXX_RspOutComm_Md1_RspOutComm_read : Inport
  MdXX_RspOutComm_Md10_RspOutComm_read : Inport  Port=2
  MdXX_RspOutComm_Md11_RspOutComm_read : Inport  Port=3
  MdXX_RspOutComm_Md12_RspOutComm_read : Inport  Port=4
  MdXX_RspOutComm_Md13_RspOutComm_read : Inport  Port=5
  MdXX_RspOutComm_Md14_RspOutComm_read : Inport  Port=6
  MdXX_RspOutComm_Md15_RspOutComm_read : Inport  Port=7
  MdXX_RspOutComm_Md16_RspOutComm_read : Inport  Port=8
  MdXX_RspOutComm_Md17_RspOutComm_read : Inport  Port=9
  MdXX_RspOutComm_Md18_RspOutComm_read : Inport  Port=10
  MdXX_RspOutComm_Md19_RspOutComm_read : Inport  Port=11
  MdXX_RspOutComm_Md2_RspOutComm_read : Inport  Port=12
  MdXX_RspOutComm_Md20_RspOutComm_read : Inport  Port=13
  MdXX_RspOutComm_Md21_RspOutComm_read : Inport  Port=14
  MdXX_RspOutComm_Md22_RspOutComm_read : Inport  Port=15
  MdXX_RspOutComm_Md23_RspOutComm_read : Inport  Port=16
  MdXX_RspOutComm_Md24_RspOutComm_read : Inport  Port=17
  MdXX_RspOutComm_Md25_RspOutComm_read : Inport  Port=18
  MdXX_RspOutComm_Md26_RspOutComm_read : Inport  Port=19
  MdXX_RspOutComm_Md27_RspOutComm_read : Inport  Port=20
  MdXX_RspOutComm_Md28_RspOutComm_read : Inport  Port=21
  MdXX_RspOutComm_Md29_RspOutComm_read : Inport  Port=22
  MdXX_RspOutComm_Md3_RspOutComm_read : Inport  Port=23
  MdXX_RspOutComm_Md30_RspOutComm_read : Inport  Port=24
  MdXX_RspOutComm_Md31_RspOutComm_read : Inport  Port=25
  MdXX_RspOutComm_Md32_RspOutComm_read : Inport  Port=26
  MdXX_RspOutComm_Md4_RspOutComm_read : Inport  Port=27
  MdXX_RspOutComm_Md5_RspOutComm_read : Inport  Port=28
  MdXX_RspOutComm_Md6_RspOutComm_read : Inport  Port=29
  MdXX_RspOutComm_Md7_RspOutComm_read : Inport  Port=30
  MdXX_RspOutComm_Md8_RspOutComm_read : Inport  Port=31
  MdXX_RspOutComm_Md9_RspOutComm_read : Inport  Port=32
  MdXX_SrcReqTp_Md1_SrcTp_read : Inport  Port=33
  MdXX_SrcReqTp_Md10_SrcTp_read : Inport  Port=34
  MdXX_SrcReqTp_Md11_SrcTp_read : Inport  Port=35
  MdXX_SrcReqTp_Md12_SrcTp_read : Inport  Port=36
  MdXX_SrcReqTp_Md13_SrcTp_read : Inport  Port=37
  MdXX_SrcReqTp_Md14_SrcTp_read : Inport  Port=38
  MdXX_SrcReqTp_Md15_SrcTp_read : Inport  Port=39
  MdXX_SrcReqTp_Md16_SrcTp_read : Inport  Port=40
  MdXX_SrcReqTp_Md17_SrcTp_read : Inport  Port=41
  MdXX_SrcReqTp_Md18_SrcTp_read : Inport  Port=42
  MdXX_SrcReqTp_Md19_SrcTp_read : Inport  Port=43
  MdXX_SrcReqTp_Md2_SrcTp_read : Inport  Port=44
  MdXX_SrcReqTp_Md20_SrcTp_read : Inport  Port=45
  MdXX_SrcReqTp_Md21_SrcTp_read : Inport  Port=46
  MdXX_SrcReqTp_Md22_SrcTp_read : Inport  Port=47
  MdXX_SrcReqTp_Md23_SrcTp_read : Inport  Port=48
  MdXX_SrcReqTp_Md24_SrcTp_read : Inport  Port=49
  MdXX_SrcReqTp_Md25_SrcTp_read : Inport  Port=50
  MdXX_SrcReqTp_Md26_SrcTp_read : Inport  Port=51
  MdXX_SrcReqTp_Md27_SrcTp_read : Inport  Port=52
  MdXX_SrcReqTp_Md28_SrcTp_read : Inport  Port=53
  MdXX_SrcReqTp_Md29_SrcTp_read : Inport  Port=54
  MdXX_SrcReqTp_Md3_SrcTp_read : Inport  Port=55
  MdXX_SrcReqTp_Md30_SrcTp_read : Inport  Port=56
  MdXX_SrcReqTp_Md31_SrcTp_read : Inport  Port=57
  MdXX_SrcReqTp_Md32_SrcTp_read : Inport  Port=58
  MdXX_SrcReqTp_Md4_SrcTp_read : Inport  Port=59
  MdXX_SrcReqTp_Md5_SrcTp_read : Inport  Port=60
  MdXX_SrcReqTp_Md6_SrcTp_read : Inport  Port=61
  MdXX_SrcReqTp_Md7_SrcTp_read : Inport  Port=62
  MdXX_SrcReqTp_Md8_SrcTp_read : Inport  Port=63
  MdXX_SrcReqTp_Md9_SrcTp_read : Inport  Port=64
  All32in1 : Subsystem
  Constant6 : Constant  Value=SrcReqTp1.SrcReqTp_SRS  OutDataTypeStr=Enum:SrcReqTp1
  Ground{,1..11} (12 alike) : Ground
  PA_KeSMSuRspStatHldTm_Val : Constant  Value=KeSMSuRspStatHldTm_Val
  RspforSrcMd{1..20} (20 alike) : RspLib/RspforSrc  SystemSampleTime=-1
  Terminator_{14..22,24..26,46..54,56..58} (24 alike) : Terminator
  IfVeSMStPassCmprtMd_RfCtrl_Sw_RclRspStat_Val_write : Outport
      settings: EnsureOutportIsVirtual=on
  wires:
  MdXX_RspOutComm_Md24_RspOutComm_read/1 -> Terminator_17/1
  MdXX_SrcReqTp_Md27_SrcTp_read/1 -> Terminator_52/1
  MdXX_SrcReqTp_Md22_SrcTp_read/1 -> Terminator_47/1
  MdXX_SrcReqTp_Md29_SrcTp_read/1 -> Terminator_54/1
  MdXX_SrcReqTp_Md31_SrcTp_read/1 -> Terminator_57/1
  MdXX_RspOutComm_Md28_RspOutComm_read/1 -> Terminator_21/1
  PA_KeSMSuRspStatHldTm_Val/1 -> [KeSMSuRspStatHldTm_Val]
  MdXX_SrcReqTp_Md32_SrcTp_read/1 -> Terminator_58/1
  MdXX_RspOutComm_Md27_RspOutComm_read/1 -> Terminator_20/1
  MdXX_RspOutComm_Md1_RspOutComm_read/1 -> RspforSrcMd1/1
  MdXX_SrcReqTp_Md21_SrcTp_read/1 -> Terminator_46/1
  MdXX_SrcReqTp_Md26_SrcTp_read/1 -> Terminator_51/1
  MdXX_RspOutComm_Md31_RspOutComm_read/1 -> Terminator_25/1
  MdXX_SrcReqTp_Md30_SrcTp_read/1 -> Terminator_56/1
  MdXX_RspOutComm_Md21_RspOutComm_read/1 -> Terminator_14/1
  MdXX_RspOutComm_Md23_RspOutComm_read/1 -> Terminator_16/1
  MdXX_RspOutComm_Md29_RspOutComm_read/1 -> Terminator_22/1
  MdXX_SrcReqTp_Md28_SrcTp_read/1 -> Terminator_53/1
  MdXX_RspOutComm_Md25_RspOutComm_read/1 -> Terminator_18/1
  MdXX_RspOutComm_Md22_RspOutComm_read/1 -> Terminator_15/1
  MdXX_SrcReqTp_Md25_SrcTp_read/1 -> Terminator_50/1
  MdXX_RspOutComm_Md32_RspOutComm_read/1 -> Terminator_26/1
  MdXX_RspOutComm_Md30_RspOutComm_read/1 -> Terminator_24/1
  MdXX_SrcReqTp_Md24_SrcTp_read/1 -> Terminator_49/1
  MdXX_RspOutComm_Md26_RspOutComm_read/1 -> Terminator_19/1
  MdXX_SrcReqTp_Md23_SrcTp_read/1 -> Terminator_48/1
  All32in1/1(Allin1Rsp) -> IfVeSMStPassCmprtMd_RfCtrl_Sw_RclRspStat_Val_write/1
  Constant6/1 -> [TargtSrc]
  [TargtSrc] -> RspforSrcMd1/3
  [KeSMSuRspStatHldTm_Val] -> RspforSrcMd1/4
  [KeSMSuRspStatHldTm_Val] -> RspforSrcMd2/4
  [TargtSrc] -> RspforSrcMd2/3
  [TargtSrc] -> RspforSrcMd3/3
  [KeSMSuRspStatHldTm_Val] -> RspforSrcMd3/4
  [KeSMSuRspStatHldTm_Val] -> RspforSrcMd4/4
  [TargtSrc] -> RspforSrcMd4/3
  [TargtSrc] -> RspforSrcMd5/3
  [KeSMSuRspStatHldTm_Val] -> RspforSrcMd5/4
  [KeSMSuRspStatHldTm_Val] -> RspforSrcMd6/4
  [TargtSrc] -> RspforSrcMd6/3
  [TargtSrc] -> RspforSrcMd7/3
  [KeSMSuRspStatHldTm_Val] -> RspforSrcMd7/4
  [KeSMSuRspStatHldTm_Val] -> RspforSrcMd8/4
  [TargtSrc] -> RspforSrcMd8/3
  [TargtSrc] -> RspforSrcMd9/3
  [KeSMSuRspStatHldTm_Val] -> RspforSrcMd9/4
  [KeSMSuRspStatHldTm_Val] -> RspforSrcMd10/4
  [TargtSrc] -> RspforSrcMd10/3
  [TargtSrc] -> RspforSrcMd11/3
  [KeSMSuRspStatHldTm_Val] -> RspforSrcMd11/4
  [KeSMSuRspStatHldTm_Val] -> RspforSrcMd12/4
  [TargtSrc] -> RspforSrcMd12/3
  [TargtSrc] -> RspforSrcMd13/3
  [KeSMSuRspStatHldTm_Val] -> RspforSrcMd13/4
  [KeSMSuRspStatHldTm_Val] -> RspforSrcMd14/4
  [TargtSrc] -> RspforSrcMd14/3
  [TargtSrc] -> RspforSrcMd15/3
  [KeSMSuRspStatHldTm_Val] -> RspforSrcMd15/4
  [KeSMSuRspStatHldTm_Val] -> RspforSrcMd16/4
  [TargtSrc] -> RspforSrcMd16/3
  [TargtSrc] -> RspforSrcMd17/3
  [KeSMSuRspStatHldTm_Val] -> RspforSrcMd17/4
  [KeSMSuRspStatHldTm_Val] -> RspforSrcMd18/4
  [TargtSrc] -> RspforSrcMd18/3
  [TargtSrc] -> RspforSrcMd19/3
  [KeSMSuRspStatHldTm_Val] -> RspforSrcMd19/4
  [KeSMSuRspStatHldTm_Val] -> RspforSrcMd20/4
  [TargtSrc] -> RspforSrcMd20/3
  RspforSrcMd1/1 -> [Md1Rsp]
  RspforSrcMd2/1 -> [Md2Rsp]
  RspforSrcMd3/1 -> [Md3Rsp]
  RspforSrcMd4/1 -> [Md4Rsp]
  RspforSrcMd5/1 -> [Md5Rsp]
  RspforSrcMd6/1 -> [Md6Rsp]
  RspforSrcMd7/1 -> [Md7Rsp]
  RspforSrcMd8/1 -> [Md8Rsp]
  RspforSrcMd9/1 -> [Md9Rsp]
  RspforSrcMd10/1 -> [Md10Rsp]
  RspforSrcMd11/1 -> [Md11Rsp]
  RspforSrcMd12/1 -> [Md12Rsp]
  RspforSrcMd13/1 -> [Md13Rsp]
  RspforSrcMd14/1 -> [Md14Rsp]
  RspforSrcMd15/1 -> [Md15Rsp]
  RspforSrcMd16/1 -> [Md16Rsp]
  RspforSrcMd17/1 -> [Md17Rsp]
  RspforSrcMd18/1 -> [Md18Rsp]
  RspforSrcMd19/1 -> [Md19Rsp]
  RspforSrcMd20/1 -> [Md20Rsp]
  [Md1Rsp] -> All32in1/1(Md1Rsp)
  [Md2Rsp] -> All32in1/2(Md2Rsp)
  [Md3Rsp] -> All32in1/3(Md3Rsp)
  [Md4Rsp] -> All32in1/4(Md4Rsp)
  [Md5Rsp] -> All32in1/5(Md5Rsp)
  [Md6Rsp] -> All32in1/6(Md6Rsp)
  [Md7Rsp] -> All32in1/7(Md7Rsp)
  [Md8Rsp] -> All32in1/8(Md8Rsp)
  [Md9Rsp] -> All32in1/9(Md9Rsp)
  [Md10Rsp] -> All32in1/10(Md10Rsp)
  [Md11Rsp] -> All32in1/11(Md11Rsp)
  [Md12Rsp] -> All32in1/12(Md12Rsp)
  [Md13Rsp] -> All32in1/13(Md13Rsp)
  [Md14Rsp] -> All32in1/14(Md14Rsp)
  [Md15Rsp] -> All32in1/15(Md15Rsp)
  [Md16Rsp] -> All32in1/16(Md16Rsp)
  [Md17Rsp] -> All32in1/17(Md17Rsp)
  [Md18Rsp] -> All32in1/18(Md18Rsp)
  [Md19Rsp] -> All32in1/19(Md19Rsp)
  [Md20Rsp] -> All32in1/20(Md20Rsp)
  Ground/1 -> All32in1/21(Md21Rsp)
  Ground1/1 -> All32in1/22(Md22Rsp)
  Ground2/1 -> All32in1/23(Md23Rsp)
  Ground3/1 -> All32in1/24(Md24Rsp)
  Ground4/1 -> All32in1/25(Md25Rsp)
  Ground5/1 -> All32in1/26(Md26Rsp)
  Ground6/1 -> All32in1/27(Md27Rsp)
  Ground7/1 -> All32in1/28(Md28Rsp)
  Ground8/1 -> All32in1/29(Md29Rsp)
  Ground9/1 -> All32in1/30(Md30Rsp)
  Ground10/1 -> All32in1/31(Md31Rsp)
  Ground11/1 -> All32in1/32(Md32Rsp)
  MdXX_RspOutComm_Md2_RspOutComm_read/1 -> RspforSrcMd2/1
  MdXX_RspOutComm_Md3_RspOutComm_read/1 -> RspforSrcMd3/1
  MdXX_RspOutComm_Md4_RspOutComm_read/1 -> RspforSrcMd4/1
  MdXX_RspOutComm_Md5_RspOutComm_read/1 -> RspforSrcMd5/1
  MdXX_RspOutComm_Md6_RspOutComm_read/1 -> RspforSrcMd6/1
  MdXX_RspOutComm_Md7_RspOutComm_read/1 -> RspforSrcMd7/1
  MdXX_RspOutComm_Md8_RspOutComm_read/1 -> RspforSrcMd8/1
  MdXX_RspOutComm_Md9_RspOutComm_read/1 -> RspforSrcMd9/1
  MdXX_SrcReqTp_Md3_SrcTp_read/1 -> RspforSrcMd3/2
  MdXX_SrcReqTp_Md4_SrcTp_read/1 -> RspforSrcMd4/2
  MdXX_SrcReqTp_Md5_SrcTp_read/1 -> RspforSrcMd5/2
  MdXX_SrcReqTp_Md6_SrcTp_read/1 -> RspforSrcMd6/2
  MdXX_SrcReqTp_Md7_SrcTp_read/1 -> RspforSrcMd7/2
  MdXX_SrcReqTp_Md8_SrcTp_read/1 -> RspforSrcMd8/2
  MdXX_SrcReqTp_Md9_SrcTp_read/1 -> RspforSrcMd9/2
  MdXX_RspOutComm_Md10_RspOutComm_read/1 -> RspforSrcMd10/1
  MdXX_SrcReqTp_Md10_SrcTp_read/1 -> RspforSrcMd10/2
  MdXX_RspOutComm_Md11_RspOutComm_read/1 -> RspforSrcMd11/1
  MdXX_SrcReqTp_Md11_SrcTp_read/1 -> RspforSrcMd11/2
  MdXX_RspOutComm_Md12_RspOutComm_read/1 -> RspforSrcMd12/1
  MdXX_SrcReqTp_Md12_SrcTp_read/1 -> RspforSrcMd12/2
  MdXX_RspOutComm_Md13_RspOutComm_read/1 -> RspforSrcMd13/1
  MdXX_SrcReqTp_Md13_SrcTp_read/1 -> RspforSrcMd13/2
  MdXX_RspOutComm_Md14_RspOutComm_read/1 -> RspforSrcMd14/1
  MdXX_SrcReqTp_Md14_SrcTp_read/1 -> RspforSrcMd14/2
  MdXX_RspOutComm_Md15_RspOutComm_read/1 -> RspforSrcMd15/1
  MdXX_SrcReqTp_Md15_SrcTp_read/1 -> RspforSrcMd15/2
  MdXX_RspOutComm_Md16_RspOutComm_read/1 -> RspforSrcMd16/1
  MdXX_SrcReqTp_Md16_SrcTp_read/1 -> RspforSrcMd16/2
  MdXX_RspOutComm_Md17_RspOutComm_read/1 -> RspforSrcMd17/1
  MdXX_SrcReqTp_Md17_SrcTp_read/1 -> RspforSrcMd17/2
  MdXX_RspOutComm_Md18_RspOutComm_read/1 -> RspforSrcMd18/1
  MdXX_SrcReqTp_Md18_SrcTp_read/1 -> RspforSrcMd18/2
  MdXX_RspOutComm_Md19_RspOutComm_read/1 -> RspforSrcMd19/1
  MdXX_SrcReqTp_Md19_SrcTp_read/1 -> RspforSrcMd19/2
  MdXX_RspOutComm_Md20_RspOutComm_read/1 -> RspforSrcMd20/1
  MdXX_SrcReqTp_Md20_SrcTp_read/1 -> RspforSrcMd20/2
  MdXX_SrcReqTp_Md1_SrcTp_read/1 -> RspforSrcMd1/2
  MdXX_SrcReqTp_Md2_SrcTp_read/1 -> RspforSrcMd2/2

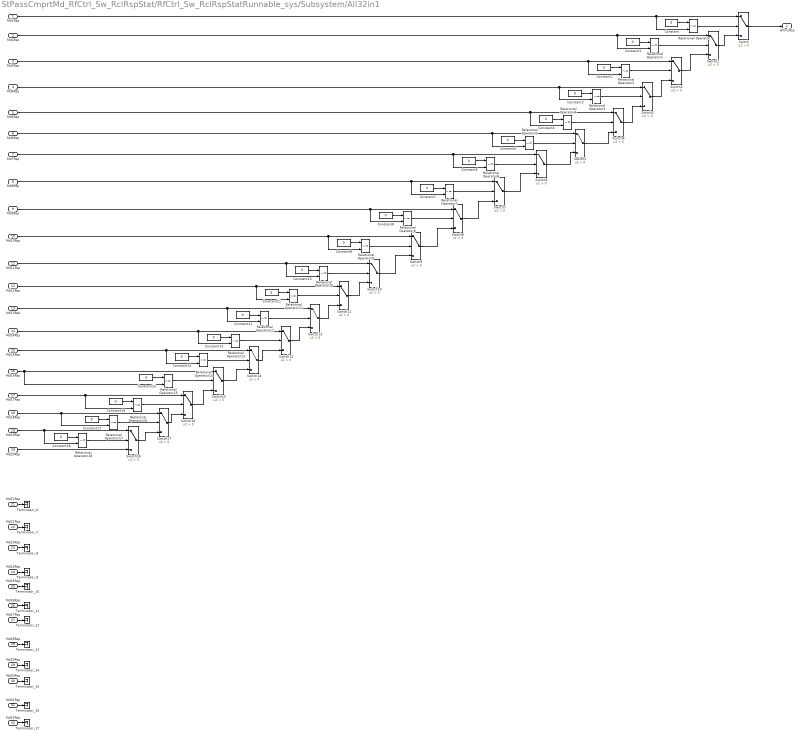
== system StPassCmprtMd_RfCtrl_Sw_RclRspStat/RfCtrl_Sw_RclRspStatRunnable_sys/Subsystem/All32in1 ==
  Md1Rsp : Inport
  Md2Rsp : Inport  Port=2
  Md3Rsp : Inport  Port=3
  Md4Rsp : Inport  Port=4
  Md5Rsp : Inport  Port=5
  Md6Rsp : Inport  Port=6
  Md7Rsp : Inport  Port=7
  Md8Rsp : Inport  Port=8
  Md9Rsp : Inport  Port=9
  Md10Rsp : Inport  Port=10
  Md11Rsp : Inport  Port=11
  Md12Rsp : Inport  Port=12
  Md13Rsp : Inport  Port=13
  Md14Rsp : Inport  Port=14
  Md15Rsp : Inport  Port=15
  Md16Rsp : Inport  Port=16
  Md17Rsp : Inport  Port=17
  Md18Rsp : Inport  Port=18
  Md19Rsp : Inport  Port=19
  Md20Rsp : Inport  Port=20
  Md21Rsp : Inport  Port=21
  Md22Rsp : Inport  Port=22
  Md23Rsp : Inport  Port=23
  Md24Rsp : Inport  Port=24
  Md25Rsp : Inport  Port=25
  Md26Rsp : Inport  Port=26
  Md27Rsp : Inport  Port=27
  Md28Rsp : Inport  Port=28
  Md29Rsp : Inport  Port=29
  Md30Rsp : Inport  Port=30
  Md31Rsp : Inport  Port=31
  Md32Rsp : Inport  Port=32
  Constant{,1..18} (19 alike) : Constant  Value=0  OutDataTypeStr=uint8
  Relational Operator{,1..18} (19 alike) : RelationalOperator  Operator=~=  OutDataTypeStr=boolean  RndMeth=Simplest
  Switch{,1..18} (19 alike) : Switch  Criteria=u2 > Threshold
  Terminator_{6..17} (12 alike) : Terminator
  Allin1Rsp : Outport
  wires:
  Md1Rsp/1 -> Relational Operator/2, Switch/1
  Constant/1 -> Relational Operator/1
  Relational Operator/1 -> Switch/2
  Switch/1 -> Allin1Rsp/1
  Switch1/1 -> Switch/3
  Relational Operator1/1 -> Switch1/2
  Constant1/1 -> Relational Operator1/1
  Md2Rsp/1 -> Relational Operator1/2, Switch1/1
  Md3Rsp/1 -> Relational Operator2/2, Switch2/1
  Constant2/1 -> Relational Operator2/1
  Relational Operator2/1 -> Switch2/2
  Switch2/1 -> Switch1/3
  Switch3/1 -> Switch2/3
  Relational Operator3/1 -> Switch3/2
  Constant3/1 -> Relational Operator3/1
  Md4Rsp/1 -> Relational Operator3/2, Switch3/1
  Md5Rsp/1 -> Relational Operator4/2, Switch4/1
  Constant4/1 -> Relational Operator4/1
  Relational Operator4/1 -> Switch4/2
  Switch4/1 -> Switch3/3
  Relational Operator5/1 -> Switch5/2
  Constant5/1 -> Relational Operator5/1
  Md6Rsp/1 -> Relational Operator5/2, Switch5/1
  Switch5/1 -> Switch4/3
  Switch6/1 -> Switch5/3
  Md7Rsp/1 -> Relational Operator6/2, Switch6/1
  Constant6/1 -> Relational Operator6/1
  Relational Operator6/1 -> Switch6/2
  Relational Operator7/1 -> Switch7/2
  Constant7/1 -> Relational Operator7/1
  Md8Rsp/1 -> Relational Operator7/2, Switch7/1
  Switch7/1 -> Switch6/3
  Switch8/1 -> Switch7/3
  Md9Rsp/1 -> Relational Operator8/2, Switch8/1
  Constant8/1 -> Relational Operator8/1
  Relational Operator8/1 -> Switch8/2
  Relational Operator9/1 -> Switch9/2
  Constant9/1 -> Relational Operator9/1
  Md10Rsp/1 -> Relational Operator9/2, Switch9/1
  Switch9/1 -> Switch8/3
  Switch10/1 -> Switch9/3
  Md11Rsp/1 -> Relational Operator10/2, Switch10/1
  Constant10/1 -> Relational Operator10/1
  Relational Operator10/1 -> Switch10/2
  Relational Operator11/1 -> Switch11/2
  Constant11/1 -> Relational Operator11/1
  Md12Rsp/1 -> Relational Operator11/2, Switch11/1
  Switch11/1 -> Switch10/3
  Switch12/1 -> Switch11/3
  Md13Rsp/1 -> Relational Operator12/2, Switch12/1
  Constant12/1 -> Relational Operator12/1
  Relational Operator12/1 -> Switch12/2
  Relational Operator13/1 -> Switch13/2
  Constant13/1 -> Relational Operator13/1
  Md14Rsp/1 -> Relational Operator13/2, Switch13/1
  Switch13/1 -> Switch12/3
  Md21Rsp/1 -> Terminator_6/1
  Md22Rsp/1 -> Terminator_7/1
  Md23Rsp/1 -> Terminator_8/1
  Md24Rsp/1 -> Terminator_9/1
  Md25Rsp/1 -> Terminator_10/1
  Md26Rsp/1 -> Terminator_11/1
  Md27Rsp/1 -> Terminator_12/1
  Md28Rsp/1 -> Terminator_13/1
  Md29Rsp/1 -> Terminator_14/1
  Md30Rsp/1 -> Terminator_15/1
  Md31Rsp/1 -> Terminator_16/1
  Md32Rsp/1 -> Terminator_17/1
  Switch15/1 -> Switch14/3
  Md15Rsp/1 -> Switch14/1, Relational Operator14/2
  Constant14/1 -> Relational Operator14/1
  Relational Operator14/1 -> Switch14/2
  Switch14/1 -> Switch13/3
  Md16Rsp/1 -> Switch15/1, Relational Operator15/2
  Relational Operator15/1 -> Switch15/2
  Constant15/1 -> Relational Operator15/1
  Switch16/1 -> Switch15/3
  Switch17/1 -> Switch16/3
  Constant16/1 -> Relational Operator16/1
  Relational Operator16/1 -> Switch16/2
  Md17Rsp/1 -> Relational Operator16/2, Switch16/1
  Md18Rsp/1 -> Switch17/1, Relational Operator17/2
  Relational Operator17/1 -> Switch17/2
  Constant17/1 -> Relational Operator17/1
  Md20Rsp/1 -> Switch18/3
  Constant18/1 -> Relational Operator18/1
  Relational Operator18/1 -> Switch18/2
  Md19Rsp/1 -> Relational Operator18/2, Switch18/1
  Switch18/1 -> Switch17/3
